simulink model "ass3q4Control"  (R2025a)
settings: Solver=VariableStepAuto  StartTime=0.0  StopTime=1200  RelTol=1e-3
values from neighbouring files (symbols this model uses):
  B = zeros(nbus)    [dc_scopf.m]    (also in dcpf.m = sparse(nbus, nbus); decpf.m = imag(Y); fastdecpf.m = imag(Y); nrpf.m = imag(Y))
  D = 20 / ( 2 * pi)    (= 3.18309886184)    [assignement_3_simulink_q1.m]    (also in ecse563_part1c_model.m)
  M = length(nfrom)    [admittance.m]    (also in assignement_3_simulink_q1.m = 111.41; ecse563_part1c_model.m = 111.4; nrpf.m = zeros(nb, nb))
  R1 = 0.0060 * 2 * pi    (= 0.0376991118431)    [assignement_3_simulink_q1.m]
  R2 = 0.0120 * 2 * pi    (= 0.0753982236862)    [assignement_3_simulink_q1.m]
  Tch1 = 3    [assignement_3_simulink_q1.m]
  Tch2 = 8    [assignement_3_simulink_q1.m]
  Tg1 = 0.25    [assignement_3_simulink_q1.m]
  Tg2 = 0.50    (= 0.5)    [assignement_3_simulink_q1.m]
undefined symbols (not defined in the file or in its folder): K, T
settings Model: Creator=aliseifeldin  LastModifiedBy=aliseifeldin

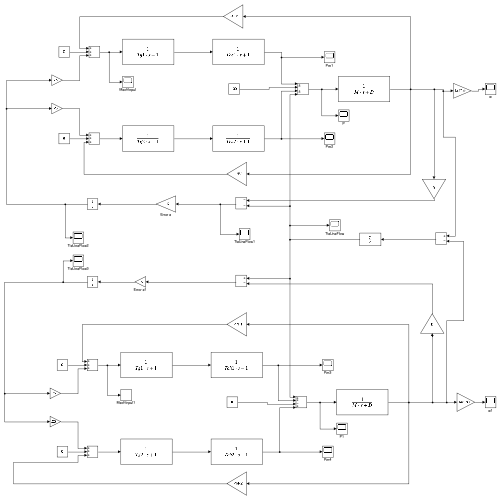
[thumbnail: Simulink's stored preview of the top-level diagram]
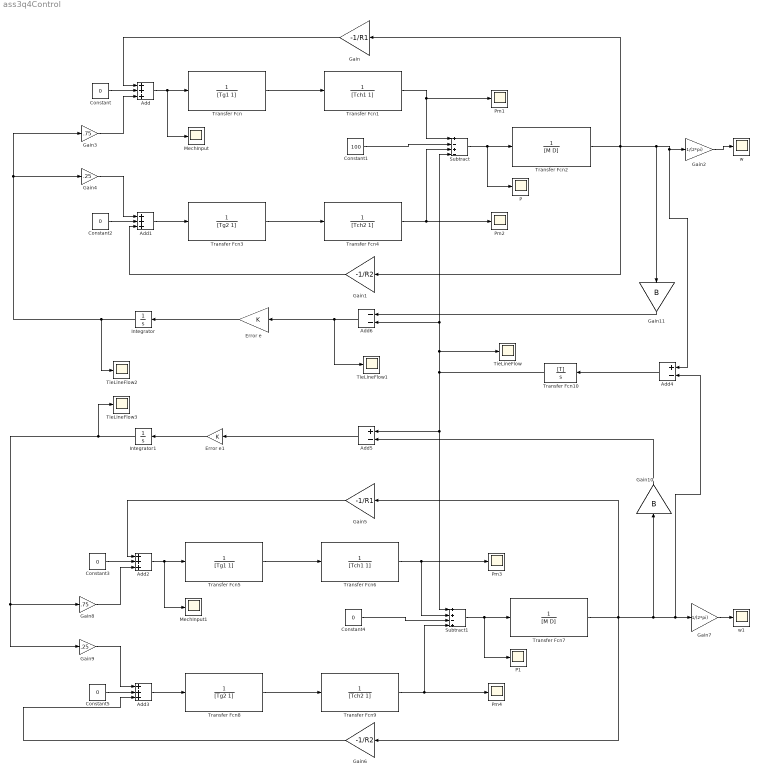
== system ass3q4Control ==
  Add{,1..3} (4 alike) : Sum  Inputs=+++
  Add4 : Sum  Inputs=+-
  Add5 : Sum  Inputs=+-
  Add6 : Sum  Inputs=--
  Constant{,2..5} (5 alike) : Constant  Value=0
  Constant1 : Constant  Value=100
  Error e : Gain  Gain=K
  Error e1 : Gain  Gain=K
  Gain : Gain  Gain=-1/R1
  Gain1 : Gain  Gain=-1/R2
  Gain10 : Gain  Gain=B
  Gain11 : Gain  Gain=B
  Gain2 : Gain  Gain=1/(2*pi)
  Gain3 : Gain  Gain=.75
  Gain4 : Gain  Gain=.25
  Gain5 : Gain  Gain=-1/R1
  Gain6 : Gain  Gain=-1/R2
  Gain7 : Gain  Gain=1/(2*pi)
  Gain8 : Gain  Gain=.75
  Gain9 : Gain  Gain=.25
  Integrator : Integrator
  Integrator1 : Integrator
  MechInput : Scope
      settings: ActiveDisplayYMinimum=-1  ActiveDisplayYMaximum=1  DataLoggingVariableName=Pm1Scope1
  MechInput1 : Scope
      settings: ActiveDisplayYMinimum=-10.410800299026624  ActiveDisplayYMaximum=93.697202691239625  DataLoggingVariableName=Pm1Scope2
  P : Scope
      settings: ActiveDisplayYMinimum=-1  ActiveDisplayYMaximum=1  DataLoggingVariableName=PScope
  P1 : Scope
      settings: ActiveDisplayYMinimum=-1  ActiveDisplayYMaximum=1  DataLoggingVariableName=PScope1
  Pm{1..4} (4 alike) : Scope
      Pm1 settings: ActiveDisplayYMinimum=-1  ActiveDisplayYMaximum=1  DataLoggingVariableName=Pm1Scope
      Pm2 settings: ActiveDisplayYMinimum=-1  ActiveDisplayYMaximum=1  DataLoggingVariableName=Pm2Scope
      Pm3 settings: ActiveDisplayYMinimum=-1  ActiveDisplayYMaximum=1  DataLoggingVariableName=Pm1Scope3
      Pm4 settings: ActiveDisplayYMinimum=-3.9741691062345192  ActiveDisplayYMaximum=35.767521956110684  DataLoggingVariableName=Pm2Scope1
  Subtract : Sum  Inputs=+-+-
  Subtract1 : Sum  Inputs=++-+
  TieLineFlow{,1..3} (4 alike) : Scope
      TieLineFlow settings: ActiveDisplayYMinimum=-115.2048655820867  ActiveDisplayYMaximum=41.904260851446942  DataLoggingVariableName=PTieLine
      TieLineFlow1 settings: ActiveDisplayYMinimum=-115.25906824846817  ActiveDisplayYMaximum=85.518397865896375  DataLoggingVariableName=PTieLine1
      TieLineFlow2 settings: ActiveDisplayYMinimum=-17.855975498765055  ActiveDisplayYMaximum=160.70377948888552  DataLoggingVariableName=PTieLine2
      TieLineFlow3 settings: ActiveDisplayYMinimum=-2.1917805509821252E+62  ActiveDisplayYMaximum=2.2771419550135088E+62  DataLoggingVariableName=PTieLine3
  Transfer Fcn : TransferFcn  Denominator=[Tg1 1]
  Transfer Fcn1 : TransferFcn  Denominator=[Tch1 1]
  Transfer Fcn10 : TransferFcn  Numerator=[T]  Denominator=[1 0]
  Transfer Fcn2 : TransferFcn  Denominator=[M D]
  Transfer Fcn3 : TransferFcn  Denominator=[Tg2 1]
  Transfer Fcn4 : TransferFcn  Denominator=[Tch2 1]
  Transfer Fcn5 : TransferFcn  Denominator=[Tg1 1]
  Transfer Fcn6 : TransferFcn  Denominator=[Tch1 1]
  Transfer Fcn7 : TransferFcn  Denominator=[M D]
  Transfer Fcn8 : TransferFcn  Denominator=[Tg2 1]
  Transfer Fcn9 : TransferFcn  Denominator=[Tch2 1]
  w : Scope
      settings: ActiveDisplayYMinimum=-0.300526113744658  ActiveDisplayYMaximum=0.12467239006965593  DataLoggingVariableName=wScope
  w1 : Scope
      settings: ActiveDisplayYMinimum=-1  ActiveDisplayYMaximum=1  DataLoggingVariableName=wScope1
  wires:
  Transfer Fcn/1 -> Transfer Fcn1/1
  Subtract/1 -> P/1, Transfer Fcn2/1
  Transfer Fcn1/1 -> Pm1/1, Subtract/1
  Transfer Fcn2/1 -> Gain1/1, Gain/1, Gain11/1, Add4/1, Gain2/1
  Gain/1 -> Add/1
  Add/1 -> MechInput/1, Transfer Fcn/1
  Constant/1 -> Add/2
  Constant1/1 -> Subtract/2
  Transfer Fcn3/1 -> Transfer Fcn4/1
  Add1/1 -> Transfer Fcn3/1
  Constant2/1 -> Add1/2
  Transfer Fcn4/1 -> Pm2/1, Subtract/3
  Gain2/1 -> w/1
  Error e/1 -> Integrator/1
  Gain1/1 -> Add1/3
  Gain4/1 -> Add1/1
  Gain3/1 -> Add/3
  Integrator/1 -> TieLineFlow2/1, Gain3/1, Gain4/1
  Transfer Fcn5/1 -> Transfer Fcn6/1
  Transfer Fcn6/1 -> Subtract1/2, Pm3/1
  Gain5/1 -> Add2/1
  Gain9/1 -> Add3/1
  Transfer Fcn8/1 -> Transfer Fcn9/1
  Gain6/1 -> Add3/3
  Gain8/1 -> Add2/3
  Transfer Fcn9/1 -> Pm4/1, Subtract1/4
  Subtract1/1 -> P1/1, Transfer Fcn7/1
  Constant5/1 -> Add3/2
  Error e1/1 -> Integrator1/1
  Gain7/1 -> w1/1
  Constant3/1 -> Add2/2
  Add2/1 -> MechInput1/1, Transfer Fcn5/1
  Add3/1 -> Transfer Fcn8/1
  Integrator1/1 -> TieLineFlow3/1, Gain9/1, Gain8/1
  Add4/1 -> Transfer Fcn10/1
  Constant4/1 -> Subtract1/3
  Transfer Fcn10/1 -> Add5/1, Subtract1/1, TieLineFlow/1, Add6/2, Subtract/4
  Transfer Fcn7/1 -> Gain6/1, Gain10/1, Add4/2, Gain7/1, Gain5/1
  Gain10/1 -> Add5/2
  Gain11/1 -> Add6/1
  Add5/1 -> Error e1/1
  Add6/1 -> TieLineFlow1/1, Error e/1
